simulink model "linear_pitch_att_control_R2015a"  (R2015a)
settings: Solver=ode45  StartTime=0.0  StopTime=10.0  RelTol=1e-3
values from neighbouring files (symbols this model uses):
  kd = 7    [RunSimLab7.m]    (also in RunSimLab7[Conflict].m)
  ki = -9    [RunSimLab7.m]    (also in RunSimLab7[Conflict].m)
  kp = -2    [RunSimLab7.m]    (also in RunSimLab7[Conflict].m)
  numP = numP(4,:)    [RunSimLab7.m]    (also in RunSimLab7[Conflict].m)
  theta_com = .5*pi/180    (= 0.00872664625997)    [RunSimLab7.m]    (also in RunSimLab7[Conflict].m)
undefined symbols (not defined in the file or in its folder): denP
settings Model: CovSFcnEnable=off  Creator=Eric  LastModifiedBy=paar5780
settings OptimizationCC: ExpressionDepthLimit=2147483647
settings DebuggingCC: UnderspecifiedInitializationDetection=Classic  MergeDetectMultiDrivingBlocksExec=none  SolverPrmCheckMsg=warning  StateNameClashWarn=warning

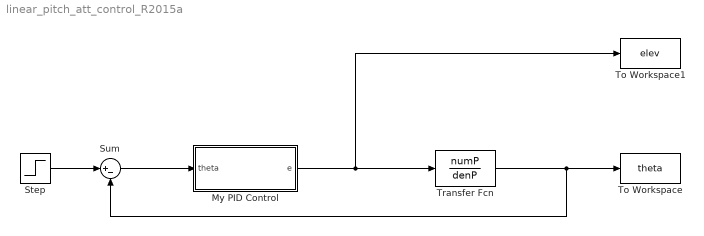
== system linear_pitch_att_control_R2015a ==
  My PID Control : Subsystem  TreatAsAtomicUnit=on
  Step : Step  Time=0  After=theta_com  SampleTime=0
  Sum : Sum  Inputs=|+-
  To Workspace : ToWorkspace  VariableName=theta  SaveFormat=Timeseries  SampleTime=-1
  To Workspace1 : ToWorkspace  VariableName=elev  SaveFormat=Timeseries  SampleTime=-1
  Transfer Fcn : TransferFcn  Numerator=numP  Denominator=denP
  wires:
  Step/1 -> Sum/1
  Sum/1 -> My PID Control/1(theta)
  My PID Control/1(e) -> To Workspace1/1, Transfer Fcn/1
  Transfer Fcn/1 -> Sum/2, To Workspace/1

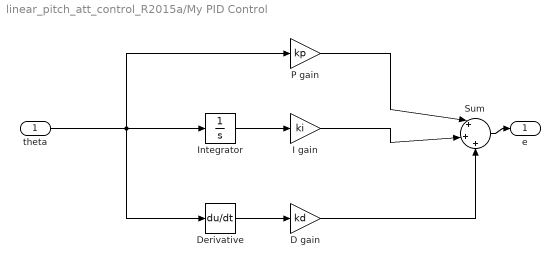
== system linear_pitch_att_control_R2015a/My PID Control ==
  theta : Inport
  D gain : Gain  Gain=kd
  Derivative : Derivative
  I gain : Gain  Gain=ki
  Integrator : Integrator
  P gain : Gain  Gain=kp
  Sum : Sum  Inputs=|+|+|+
  e : Outport
  wires:
  theta/1 -> Derivative/1, Integrator/1, P gain/1
  I gain/1 -> Sum/2
  P gain/1 -> Sum/1
  Sum/1 -> e/1
  D gain/1 -> Sum/3
  Integrator/1 -> I gain/1
  Derivative/1 -> D gain/1
